simulink model "Adder"  (R2019b)
settings: Solver=VariableStepAuto  StartTime=0.0  StopTime=10.0  RelTol=1e-3
libraries: hdlsllib x17
settings Model: Creator=cohen  LastModifiedBy=cohen

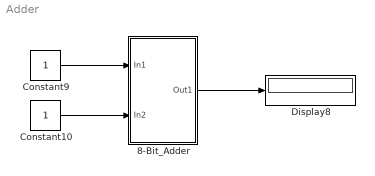
== system Adder ==
  8-Bit_Adder : Subsystem
  Constant10 : Constant  OutDataTypeStr=int8
  Constant9 : Constant  OutDataTypeStr=int8
  Display8 : Display
  wires:
  8-Bit_Adder/1(Out1) -> Display8/1
  Constant10/1 -> 8-Bit_Adder/2(In2)
  Constant9/1 -> 8-Bit_Adder/1(In1)

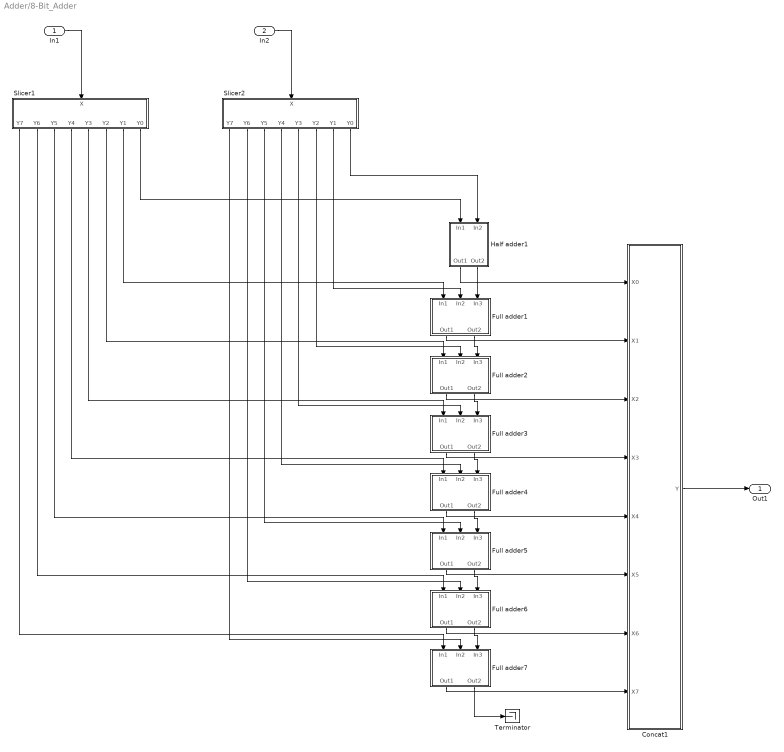
== system Adder/8-Bit_Adder ==
  In1 : Inport  OutDataTypeStr=uint8
  In2 : Inport  Port=2  OutDataTypeStr=uint8
  Concat1 : Subsystem
  Full adder1 : Subsystem
  Full adder2 : Subsystem
  Full adder3 : Subsystem
  Full adder4 : Subsystem
  Full adder5 : Subsystem
  Full adder6 : Subsystem
  Full adder7 : Subsystem
  Half adder1 : Subsystem
  Slicer1 : Subsystem
  Slicer2 : Subsystem
  Terminator : Terminator
  Out1 : Outport
  wires:
  Slicer1/7(Y1) -> Full adder1/1(In1)
  Full adder2/2(Out2) -> Full adder3/3(In3)
  Slicer1/1(Y7) -> Full adder7/1(In1)
  Full adder5/2(Out2) -> Full adder6/3(In3)
  Slicer1/4(Y4) -> Full adder4/1(In1)
  In1/1 -> Slicer1/1(X)
  Slicer1/2(Y6) -> Full adder6/1(In1)
  Full adder6/2(Out2) -> Full adder7/3(In3)
  Slicer2/4(Y4) -> Full adder4/2(In2)
  Slicer1/3(Y5) -> Full adder5/1(In1)
  Concat1/1(Y) -> Out1/1
  Full adder3/2(Out2) -> Full adder4/3(In3)
  Full adder4/2(Out2) -> Full adder5/3(In3)
  Full adder1/2(Out2) -> Full adder2/3(In3)
  Slicer2/2(Y6) -> Full adder6/2(In2)
  Slicer1/8(Y0) -> Half adder1/1(In1)
  Slicer2/3(Y5) -> Full adder5/2(In2)
  Slicer2/1(Y7) -> Full adder7/2(In2)
  Slicer1/6(Y2) -> Full adder2/1(In1)
  Half adder1/2(Out2) -> Full adder1/3(In3)
  Slicer2/5(Y3) -> Full adder3/2(In2)
  In2/1 -> Slicer2/1(X)
  Slicer2/8(Y0) -> Half adder1/2(In2)
  Slicer2/7(Y1) -> Full adder1/2(In2)
  Slicer1/5(Y3) -> Full adder3/1(In1)
  Slicer2/6(Y2) -> Full adder2/2(In2)
  Full adder7/2(Out2) -> Terminator/1
  Full adder7/1(Out1) -> Concat1/8(X7)
  Full adder6/1(Out1) -> Concat1/7(X6)
  Full adder5/1(Out1) -> Concat1/6(X5)
  Full adder4/1(Out1) -> Concat1/5(X4)
  Full adder3/1(Out1) -> Concat1/4(X3)
  Full adder2/1(Out1) -> Concat1/3(X2)
  Full adder1/1(Out1) -> Concat1/2(X1)
  Half adder1/1(Out1) -> Concat1/1(X0)

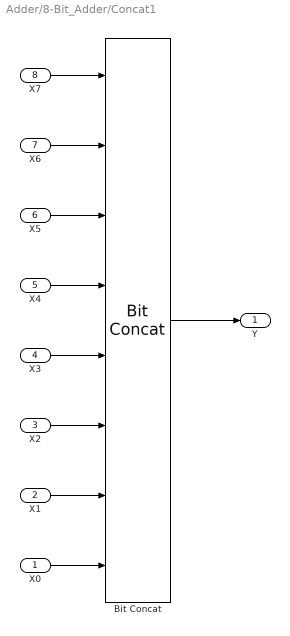
== system Adder/8-Bit_Adder/Concat1 ==
  X0 : Inport  OutDataTypeStr=boolean  SampleTime=1
  X1 : Inport  Port=2  OutDataTypeStr=boolean  SampleTime=1
  X2 : Inport  Port=3  OutDataTypeStr=boolean  SampleTime=1
  X3 : Inport  Port=4  OutDataTypeStr=boolean  SampleTime=1
  X4 : Inport  Port=5  OutDataTypeStr=boolean  SampleTime=1
  X5 : Inport  Port=6  OutDataTypeStr=boolean  SampleTime=1
  X6 : Inport  Port=7  OutDataTypeStr=boolean  SampleTime=1
  X7 : Inport  Port=8  OutDataTypeStr=boolean  SampleTime=1
  Bit Concat : hdlsllib/Logic and Bit Operations/Bit Concat  numInputs=8
      settings: SourceProductName=Simulink
  Y : Outport
  wires:
  X6/1 -> Bit Concat/2
  X2/1 -> Bit Concat/6
  X7/1 -> Bit Concat/1
  X0/1 -> Bit Concat/8
  Bit Concat/1 -> Y/1
  X3/1 -> Bit Concat/5
  X1/1 -> Bit Concat/7
  X5/1 -> Bit Concat/3
  X4/1 -> Bit Concat/4

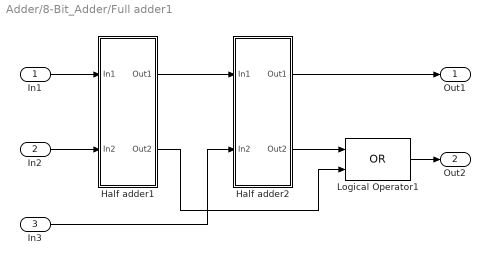
== system Adder/8-Bit_Adder/Full adder1 ==
  In1 : Inport  OutDataTypeStr=boolean
  In2 : Inport  Port=2  OutDataTypeStr=boolean
  In3 : Inport  Port=3  OutDataTypeStr=boolean
  Half adder1 : Subsystem
  Half adder2 : Subsystem
  Logical Operator1 : Logic  Operator=OR  AllPortsSameDT=off  OutDataTypeStr=boolean
  Out1 : Outport
  Out2 : Outport  Port=2
  wires:
  Logical Operator1/1 -> Out2/1
  In1/1 -> Half adder1/1(In1)
  Half adder2/1(Out1) -> Out1/1
  In2/1 -> Half adder1/2(In2)
  In3/1 -> Half adder2/2(In2)
  Half adder1/2(Out2) -> Logical Operator1/2
  Half adder1/1(Out1) -> Half adder2/1(In1)
  Half adder2/2(Out2) -> Logical Operator1/1

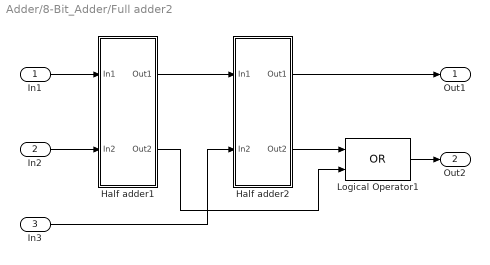
== system Adder/8-Bit_Adder/Full adder2 ==
  In1 : Inport  OutDataTypeStr=boolean
  In2 : Inport  Port=2  OutDataTypeStr=boolean
  In3 : Inport  Port=3  OutDataTypeStr=boolean
  Half adder1 : Subsystem
  Half adder2 : Subsystem
  Logical Operator1 : Logic  Operator=OR  AllPortsSameDT=off  OutDataTypeStr=boolean
  Out1 : Outport
  Out2 : Outport  Port=2
  wires:
  Logical Operator1/1 -> Out2/1
  In1/1 -> Half adder1/1(In1)
  Half adder2/1(Out1) -> Out1/1
  In2/1 -> Half adder1/2(In2)
  In3/1 -> Half adder2/2(In2)
  Half adder1/2(Out2) -> Logical Operator1/2
  Half adder1/1(Out1) -> Half adder2/1(In1)
  Half adder2/2(Out2) -> Logical Operator1/1

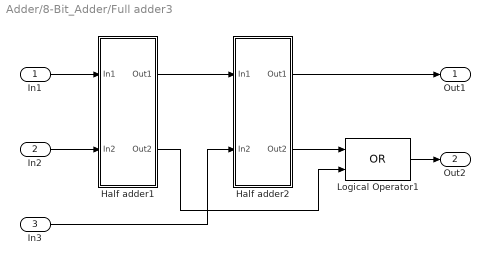
== system Adder/8-Bit_Adder/Full adder3 ==
  In1 : Inport  OutDataTypeStr=boolean
  In2 : Inport  Port=2  OutDataTypeStr=boolean
  In3 : Inport  Port=3  OutDataTypeStr=boolean
  Half adder1 : Subsystem
  Half adder2 : Subsystem
  Logical Operator1 : Logic  Operator=OR  AllPortsSameDT=off  OutDataTypeStr=boolean
  Out1 : Outport
  Out2 : Outport  Port=2
  wires:
  Logical Operator1/1 -> Out2/1
  In1/1 -> Half adder1/1(In1)
  Half adder2/1(Out1) -> Out1/1
  In2/1 -> Half adder1/2(In2)
  In3/1 -> Half adder2/2(In2)
  Half adder1/2(Out2) -> Logical Operator1/2
  Half adder1/1(Out1) -> Half adder2/1(In1)
  Half adder2/2(Out2) -> Logical Operator1/1

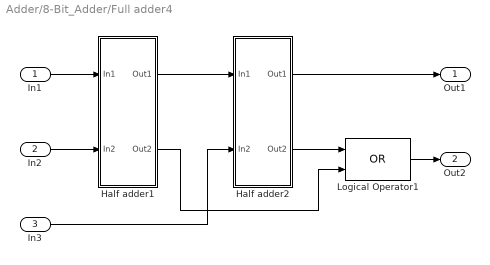
== system Adder/8-Bit_Adder/Full adder4 ==
  In1 : Inport  OutDataTypeStr=boolean
  In2 : Inport  Port=2  OutDataTypeStr=boolean
  In3 : Inport  Port=3  OutDataTypeStr=boolean
  Half adder1 : Subsystem
  Half adder2 : Subsystem
  Logical Operator1 : Logic  Operator=OR  AllPortsSameDT=off  OutDataTypeStr=boolean
  Out1 : Outport
  Out2 : Outport  Port=2
  wires:
  Logical Operator1/1 -> Out2/1
  In1/1 -> Half adder1/1(In1)
  Half adder2/1(Out1) -> Out1/1
  In2/1 -> Half adder1/2(In2)
  In3/1 -> Half adder2/2(In2)
  Half adder1/2(Out2) -> Logical Operator1/2
  Half adder1/1(Out1) -> Half adder2/1(In1)
  Half adder2/2(Out2) -> Logical Operator1/1

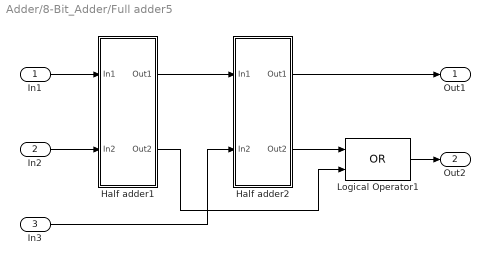
== system Adder/8-Bit_Adder/Full adder5 ==
  In1 : Inport  OutDataTypeStr=boolean
  In2 : Inport  Port=2  OutDataTypeStr=boolean
  In3 : Inport  Port=3  OutDataTypeStr=boolean
  Half adder1 : Subsystem
  Half adder2 : Subsystem
  Logical Operator1 : Logic  Operator=OR  AllPortsSameDT=off  OutDataTypeStr=boolean
  Out1 : Outport
  Out2 : Outport  Port=2
  wires:
  Logical Operator1/1 -> Out2/1
  In1/1 -> Half adder1/1(In1)
  Half adder2/1(Out1) -> Out1/1
  In2/1 -> Half adder1/2(In2)
  In3/1 -> Half adder2/2(In2)
  Half adder1/2(Out2) -> Logical Operator1/2
  Half adder1/1(Out1) -> Half adder2/1(In1)
  Half adder2/2(Out2) -> Logical Operator1/1

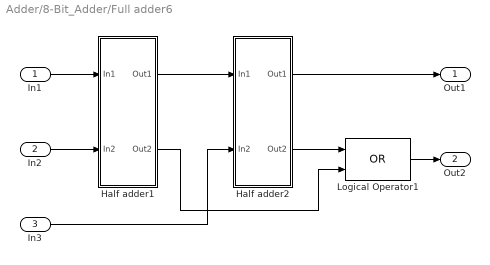
== system Adder/8-Bit_Adder/Full adder6 ==
  In1 : Inport  OutDataTypeStr=boolean
  In2 : Inport  Port=2  OutDataTypeStr=boolean
  In3 : Inport  Port=3  OutDataTypeStr=boolean
  Half adder1 : Subsystem
  Half adder2 : Subsystem
  Logical Operator1 : Logic  Operator=OR  AllPortsSameDT=off  OutDataTypeStr=boolean
  Out1 : Outport
  Out2 : Outport  Port=2
  wires:
  Logical Operator1/1 -> Out2/1
  In1/1 -> Half adder1/1(In1)
  Half adder2/1(Out1) -> Out1/1
  In2/1 -> Half adder1/2(In2)
  In3/1 -> Half adder2/2(In2)
  Half adder1/2(Out2) -> Logical Operator1/2
  Half adder1/1(Out1) -> Half adder2/1(In1)
  Half adder2/2(Out2) -> Logical Operator1/1

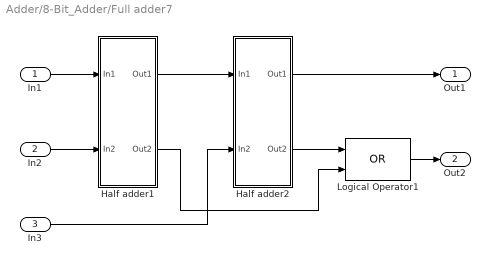
== system Adder/8-Bit_Adder/Full adder7 ==
  In1 : Inport  OutDataTypeStr=boolean
  In2 : Inport  Port=2  OutDataTypeStr=boolean
  In3 : Inport  Port=3  OutDataTypeStr=boolean
  Half adder1 : Subsystem
  Half adder2 : Subsystem
  Logical Operator1 : Logic  Operator=OR  AllPortsSameDT=off  OutDataTypeStr=boolean
  Out1 : Outport
  Out2 : Outport  Port=2
  wires:
  Logical Operator1/1 -> Out2/1
  In1/1 -> Half adder1/1(In1)
  Half adder2/1(Out1) -> Out1/1
  In2/1 -> Half adder1/2(In2)
  In3/1 -> Half adder2/2(In2)
  Half adder1/2(Out2) -> Logical Operator1/2
  Half adder1/1(Out1) -> Half adder2/1(In1)
  Half adder2/2(Out2) -> Logical Operator1/1

== system Adder/8-Bit_Adder/Half adder1 ==
  In1 : Inport  OutDataTypeStr=boolean
  In2 : Inport  Port=2  OutDataTypeStr=boolean
  Logical Operator : Logic  AllPortsSameDT=off  OutDataTypeStr=boolean
  Logical Operator1 : Logic  Operator=XOR  AllPortsSameDT=off  OutDataTypeStr=boolean
  Out1 : Outport
  Out2 : Outport  Port=2
  wires:
  In2/1 -> Logical Operator/2, Logical Operator1/2
  In1/1 -> Logical Operator/1, Logical Operator1/1
  Logical Operator1/1 -> Out1/1
  Logical Operator/1 -> Out2/1

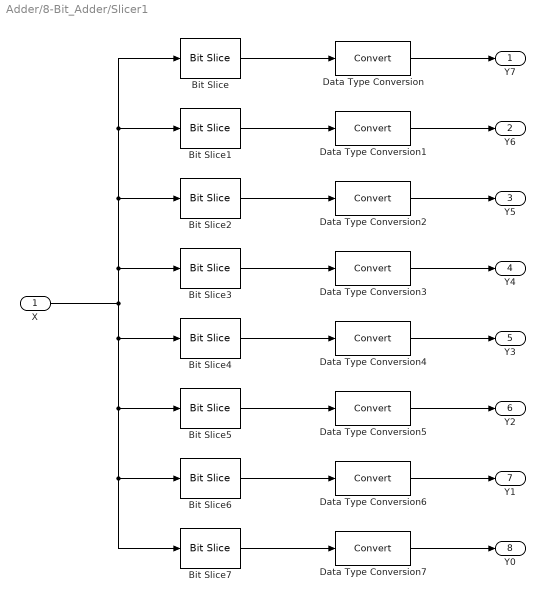
== system Adder/8-Bit_Adder/Slicer1 ==
  X : Inport  OutDataTypeStr=uint8  SampleTime=1
  Bit Slice : hdlsllib/Logic and Bit Operations/Bit Slice  lidx=7  ridx=7
      settings: SourceProductName=Simulink  SourceProductBaseCode=SL
  Bit Slice1 : hdlsllib/Logic and Bit Operations/Bit Slice  lidx=6  ridx=6
      settings: SourceProductName=Simulink  SourceProductBaseCode=SL
  Bit Slice2 : hdlsllib/Logic and Bit Operations/Bit Slice  lidx=5  ridx=5
      settings: SourceProductName=Simulink  SourceProductBaseCode=SL
  Bit Slice3 : hdlsllib/Logic and Bit Operations/Bit Slice  lidx=4  ridx=4
      settings: SourceProductName=Simulink  SourceProductBaseCode=SL
  Bit Slice4 : hdlsllib/Logic and Bit Operations/Bit Slice  lidx=3  ridx=3
      settings: SourceProductName=Simulink  SourceProductBaseCode=SL
  Bit Slice5 : hdlsllib/Logic and Bit Operations/Bit Slice  lidx=2  ridx=2
      settings: SourceProductName=Simulink  SourceProductBaseCode=SL
  Bit Slice6 : hdlsllib/Logic and Bit Operations/Bit Slice  lidx=1  ridx=1
      settings: SourceProductName=Simulink  SourceProductBaseCode=SL
  Bit Slice7 : hdlsllib/Logic and Bit Operations/Bit Slice  lidx=0  ridx=0
      settings: SourceProductName=Simulink  SourceProductBaseCode=SL
  Data Type Conversion{,1..7} (8 alike) : DataTypeConversion
  Y7 : Outport
  Y6 : Outport  Port=2
  Y5 : Outport  Port=3
  Y4 : Outport  Port=4
  Y3 : Outport  Port=5
  Y2 : Outport  Port=6
  Y1 : Outport  Port=7
  Y0 : Outport  Port=8
  wires:
  Bit Slice6/1 -> Data Type Conversion6/1
  X/1 -> Bit Slice3/1, Bit Slice2/1, Bit Slice1/1, Bit Slice/1, Bit Slice4/1, Bit Slice5/1, Bit Slice6/1, Bit Slice7/1
  Bit Slice/1 -> Data Type Conversion/1
  Bit Slice7/1 -> Data Type Conversion7/1
  Bit Slice4/1 -> Data Type Conversion4/1
  Bit Slice1/1 -> Data Type Conversion1/1
  Bit Slice3/1 -> Data Type Conversion3/1
  Data Type Conversion1/1 -> Y6/1
  Data Type Conversion7/1 -> Y0/1
  Data Type Conversion5/1 -> Y2/1
  Data Type Conversion3/1 -> Y4/1
  Data Type Conversion4/1 -> Y3/1
  Bit Slice2/1 -> Data Type Conversion2/1
  Bit Slice5/1 -> Data Type Conversion5/1
  Data Type Conversion6/1 -> Y1/1
  Data Type Conversion/1 -> Y7/1
  Data Type Conversion2/1 -> Y5/1

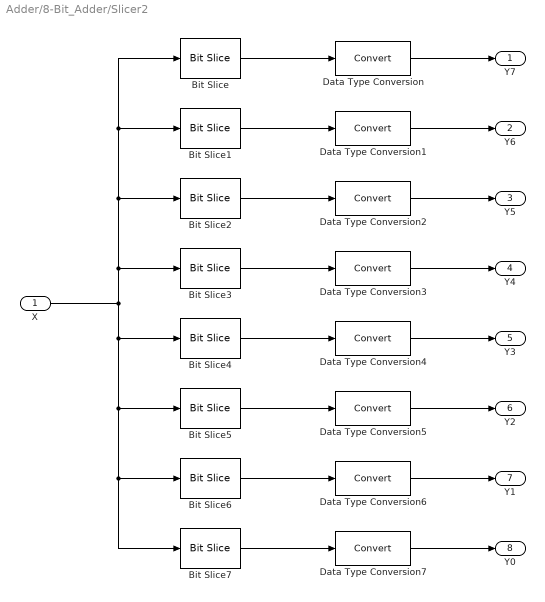
== system Adder/8-Bit_Adder/Slicer2 ==
  X : Inport  OutDataTypeStr=uint8  SampleTime=1
  Bit Slice : hdlsllib/Logic and Bit Operations/Bit Slice  lidx=7  ridx=7
      settings: SourceProductName=Simulink  SourceProductBaseCode=SL
  Bit Slice1 : hdlsllib/Logic and Bit Operations/Bit Slice  lidx=6  ridx=6
      settings: SourceProductName=Simulink  SourceProductBaseCode=SL
  Bit Slice2 : hdlsllib/Logic and Bit Operations/Bit Slice  lidx=5  ridx=5
      settings: SourceProductName=Simulink  SourceProductBaseCode=SL
  Bit Slice3 : hdlsllib/Logic and Bit Operations/Bit Slice  lidx=4  ridx=4
      settings: SourceProductName=Simulink  SourceProductBaseCode=SL
  Bit Slice4 : hdlsllib/Logic and Bit Operations/Bit Slice  lidx=3  ridx=3
      settings: SourceProductName=Simulink  SourceProductBaseCode=SL
  Bit Slice5 : hdlsllib/Logic and Bit Operations/Bit Slice  lidx=2  ridx=2
      settings: SourceProductName=Simulink  SourceProductBaseCode=SL
  Bit Slice6 : hdlsllib/Logic and Bit Operations/Bit Slice  lidx=1  ridx=1
      settings: SourceProductName=Simulink  SourceProductBaseCode=SL
  Bit Slice7 : hdlsllib/Logic and Bit Operations/Bit Slice  lidx=0  ridx=0
      settings: SourceProductName=Simulink  SourceProductBaseCode=SL
  Data Type Conversion{,1..7} (8 alike) : DataTypeConversion
  Y7 : Outport
  Y6 : Outport  Port=2
  Y5 : Outport  Port=3
  Y4 : Outport  Port=4
  Y3 : Outport  Port=5
  Y2 : Outport  Port=6
  Y1 : Outport  Port=7
  Y0 : Outport  Port=8
  wires:
  Bit Slice6/1 -> Data Type Conversion6/1
  X/1 -> Bit Slice3/1, Bit Slice2/1, Bit Slice1/1, Bit Slice/1, Bit Slice4/1, Bit Slice5/1, Bit Slice6/1, Bit Slice7/1
  Bit Slice/1 -> Data Type Conversion/1
  Bit Slice7/1 -> Data Type Conversion7/1
  Bit Slice4/1 -> Data Type Conversion4/1
  Bit Slice1/1 -> Data Type Conversion1/1
  Bit Slice3/1 -> Data Type Conversion3/1
  Data Type Conversion1/1 -> Y6/1
  Data Type Conversion7/1 -> Y0/1
  Data Type Conversion5/1 -> Y2/1
  Data Type Conversion3/1 -> Y4/1
  Data Type Conversion4/1 -> Y3/1
  Bit Slice2/1 -> Data Type Conversion2/1
  Bit Slice5/1 -> Data Type Conversion5/1
  Data Type Conversion6/1 -> Y1/1
  Data Type Conversion/1 -> Y7/1
  Data Type Conversion2/1 -> Y5/1

== system Adder/8-Bit_Adder/Full adder1/Half adder1 ==
  In1 : Inport  OutDataTypeStr=boolean
  In2 : Inport  Port=2  OutDataTypeStr=boolean
  Logical Operator : Logic  AllPortsSameDT=off  OutDataTypeStr=boolean
  Logical Operator1 : Logic  Operator=XOR  AllPortsSameDT=off  OutDataTypeStr=boolean
  Out1 : Outport
  Out2 : Outport  Port=2
  wires:
  In2/1 -> Logical Operator/2, Logical Operator1/2
  In1/1 -> Logical Operator/1, Logical Operator1/1
  Logical Operator1/1 -> Out1/1
  Logical Operator/1 -> Out2/1

== system Adder/8-Bit_Adder/Full adder1/Half adder2 ==
  In1 : Inport  OutDataTypeStr=boolean
  In2 : Inport  Port=2  OutDataTypeStr=boolean
  Logical Operator : Logic  AllPortsSameDT=off  OutDataTypeStr=boolean
  Logical Operator1 : Logic  Operator=XOR  AllPortsSameDT=off  OutDataTypeStr=boolean
  Out1 : Outport
  Out2 : Outport  Port=2
  wires:
  In2/1 -> Logical Operator/2, Logical Operator1/2
  In1/1 -> Logical Operator/1, Logical Operator1/1
  Logical Operator1/1 -> Out1/1
  Logical Operator/1 -> Out2/1

== system Adder/8-Bit_Adder/Full adder2/Half adder1 ==
  In1 : Inport  OutDataTypeStr=boolean
  In2 : Inport  Port=2  OutDataTypeStr=boolean
  Logical Operator : Logic  AllPortsSameDT=off  OutDataTypeStr=boolean
  Logical Operator1 : Logic  Operator=XOR  AllPortsSameDT=off  OutDataTypeStr=boolean
  Out1 : Outport
  Out2 : Outport  Port=2
  wires:
  In2/1 -> Logical Operator/2, Logical Operator1/2
  In1/1 -> Logical Operator/1, Logical Operator1/1
  Logical Operator1/1 -> Out1/1
  Logical Operator/1 -> Out2/1

== system Adder/8-Bit_Adder/Full adder2/Half adder2 ==
  In1 : Inport  OutDataTypeStr=boolean
  In2 : Inport  Port=2  OutDataTypeStr=boolean
  Logical Operator : Logic  AllPortsSameDT=off  OutDataTypeStr=boolean
  Logical Operator1 : Logic  Operator=XOR  AllPortsSameDT=off  OutDataTypeStr=boolean
  Out1 : Outport
  Out2 : Outport  Port=2
  wires:
  In2/1 -> Logical Operator/2, Logical Operator1/2
  In1/1 -> Logical Operator/1, Logical Operator1/1
  Logical Operator1/1 -> Out1/1
  Logical Operator/1 -> Out2/1

== system Adder/8-Bit_Adder/Full adder3/Half adder1 ==
  In1 : Inport  OutDataTypeStr=boolean
  In2 : Inport  Port=2  OutDataTypeStr=boolean
  Logical Operator : Logic  AllPortsSameDT=off  OutDataTypeStr=boolean
  Logical Operator1 : Logic  Operator=XOR  AllPortsSameDT=off  OutDataTypeStr=boolean
  Out1 : Outport
  Out2 : Outport  Port=2
  wires:
  In2/1 -> Logical Operator/2, Logical Operator1/2
  In1/1 -> Logical Operator/1, Logical Operator1/1
  Logical Operator1/1 -> Out1/1
  Logical Operator/1 -> Out2/1

== system Adder/8-Bit_Adder/Full adder3/Half adder2 ==
  In1 : Inport  OutDataTypeStr=boolean
  In2 : Inport  Port=2  OutDataTypeStr=boolean
  Logical Operator : Logic  AllPortsSameDT=off  OutDataTypeStr=boolean
  Logical Operator1 : Logic  Operator=XOR  AllPortsSameDT=off  OutDataTypeStr=boolean
  Out1 : Outport
  Out2 : Outport  Port=2
  wires:
  In2/1 -> Logical Operator/2, Logical Operator1/2
  In1/1 -> Logical Operator/1, Logical Operator1/1
  Logical Operator1/1 -> Out1/1
  Logical Operator/1 -> Out2/1

== system Adder/8-Bit_Adder/Full adder4/Half adder1 ==
  In1 : Inport  OutDataTypeStr=boolean
  In2 : Inport  Port=2  OutDataTypeStr=boolean
  Logical Operator : Logic  AllPortsSameDT=off  OutDataTypeStr=boolean
  Logical Operator1 : Logic  Operator=XOR  AllPortsSameDT=off  OutDataTypeStr=boolean
  Out1 : Outport
  Out2 : Outport  Port=2
  wires:
  In2/1 -> Logical Operator/2, Logical Operator1/2
  In1/1 -> Logical Operator/1, Logical Operator1/1
  Logical Operator1/1 -> Out1/1
  Logical Operator/1 -> Out2/1

== system Adder/8-Bit_Adder/Full adder4/Half adder2 ==
  In1 : Inport  OutDataTypeStr=boolean
  In2 : Inport  Port=2  OutDataTypeStr=boolean
  Logical Operator : Logic  AllPortsSameDT=off  OutDataTypeStr=boolean
  Logical Operator1 : Logic  Operator=XOR  AllPortsSameDT=off  OutDataTypeStr=boolean
  Out1 : Outport
  Out2 : Outport  Port=2
  wires:
  In2/1 -> Logical Operator/2, Logical Operator1/2
  In1/1 -> Logical Operator/1, Logical Operator1/1
  Logical Operator1/1 -> Out1/1
  Logical Operator/1 -> Out2/1

== system Adder/8-Bit_Adder/Full adder5/Half adder1 ==
  In1 : Inport  OutDataTypeStr=boolean
  In2 : Inport  Port=2  OutDataTypeStr=boolean
  Logical Operator : Logic  AllPortsSameDT=off  OutDataTypeStr=boolean
  Logical Operator1 : Logic  Operator=XOR  AllPortsSameDT=off  OutDataTypeStr=boolean
  Out1 : Outport
  Out2 : Outport  Port=2
  wires:
  In2/1 -> Logical Operator/2, Logical Operator1/2
  In1/1 -> Logical Operator/1, Logical Operator1/1
  Logical Operator1/1 -> Out1/1
  Logical Operator/1 -> Out2/1

== system Adder/8-Bit_Adder/Full adder5/Half adder2 ==
  In1 : Inport  OutDataTypeStr=boolean
  In2 : Inport  Port=2  OutDataTypeStr=boolean
  Logical Operator : Logic  AllPortsSameDT=off  OutDataTypeStr=boolean
  Logical Operator1 : Logic  Operator=XOR  AllPortsSameDT=off  OutDataTypeStr=boolean
  Out1 : Outport
  Out2 : Outport  Port=2
  wires:
  In2/1 -> Logical Operator/2, Logical Operator1/2
  In1/1 -> Logical Operator/1, Logical Operator1/1
  Logical Operator1/1 -> Out1/1
  Logical Operator/1 -> Out2/1

== system Adder/8-Bit_Adder/Full adder6/Half adder1 ==
  In1 : Inport  OutDataTypeStr=boolean
  In2 : Inport  Port=2  OutDataTypeStr=boolean
  Logical Operator : Logic  AllPortsSameDT=off  OutDataTypeStr=boolean
  Logical Operator1 : Logic  Operator=XOR  AllPortsSameDT=off  OutDataTypeStr=boolean
  Out1 : Outport
  Out2 : Outport  Port=2
  wires:
  In2/1 -> Logical Operator/2, Logical Operator1/2
  In1/1 -> Logical Operator/1, Logical Operator1/1
  Logical Operator1/1 -> Out1/1
  Logical Operator/1 -> Out2/1

== system Adder/8-Bit_Adder/Full adder6/Half adder2 ==
  In1 : Inport  OutDataTypeStr=boolean
  In2 : Inport  Port=2  OutDataTypeStr=boolean
  Logical Operator : Logic  AllPortsSameDT=off  OutDataTypeStr=boolean
  Logical Operator1 : Logic  Operator=XOR  AllPortsSameDT=off  OutDataTypeStr=boolean
  Out1 : Outport
  Out2 : Outport  Port=2
  wires:
  In2/1 -> Logical Operator/2, Logical Operator1/2
  In1/1 -> Logical Operator/1, Logical Operator1/1
  Logical Operator1/1 -> Out1/1
  Logical Operator/1 -> Out2/1

== system Adder/8-Bit_Adder/Full adder7/Half adder1 ==
  In1 : Inport  OutDataTypeStr=boolean
  In2 : Inport  Port=2  OutDataTypeStr=boolean
  Logical Operator : Logic  AllPortsSameDT=off  OutDataTypeStr=boolean
  Logical Operator1 : Logic  Operator=XOR  AllPortsSameDT=off  OutDataTypeStr=boolean
  Out1 : Outport
  Out2 : Outport  Port=2
  wires:
  In2/1 -> Logical Operator/2, Logical Operator1/2
  In1/1 -> Logical Operator/1, Logical Operator1/1
  Logical Operator1/1 -> Out1/1
  Logical Operator/1 -> Out2/1

== system Adder/8-Bit_Adder/Full adder7/Half adder2 ==
  In1 : Inport  OutDataTypeStr=boolean
  In2 : Inport  Port=2  OutDataTypeStr=boolean
  Logical Operator : Logic  AllPortsSameDT=off  OutDataTypeStr=boolean
  Logical Operator1 : Logic  Operator=XOR  AllPortsSameDT=off  OutDataTypeStr=boolean
  Out1 : Outport
  Out2 : Outport  Port=2
  wires:
  In2/1 -> Logical Operator/2, Logical Operator1/2
  In1/1 -> Logical Operator/1, Logical Operator1/1
  Logical Operator1/1 -> Out1/1
  Logical Operator/1 -> Out2/1
